simulink model "Project_PeregrineFalconDive_I"  (R2020b)
settings: Solver=VariableStepAuto  StartTime=0.0  StopTime=10.0  RelTol=1e-3
StartFcn:
  | learning.simulink.clearGlows(gcs);learning.simulink.resetGraderBadge(gcs);learning.simulink.closeNotificationBar(gcs);learning.simulink.Application.getInstance().clearStateflowBreakpoints()
StopFcn:
  | save_system(gcs);learning.simulink.refreshSignalWindows
model workspace (MAT data in the model file):
  courseObject.course = 'simulink'
  courseObject.chapter = 13
  courseObject.lesson = 1
  courseObject.section = 2
  courseObject.task = 1
undefined symbols (not defined in the file): A, Cd, g, m, rho
CloseFcn:
  | learning.simulink.cleanupOnlineTraining
settings Model: Creator=bhuva  LastModifiedBy=bhuva
settings DataIOCC: SaveTime=off

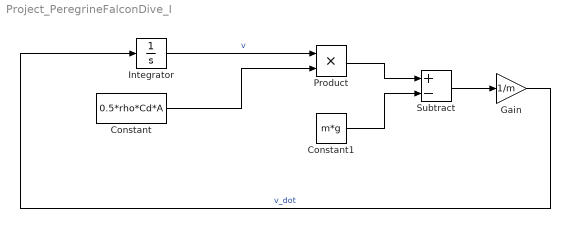
== system Project_PeregrineFalconDive_I ==
  Constant : Constant  Value=0.5*rho*Cd*A
  Constant1 : Constant  Value=m*g
  Gain : Gain  Gain=1/m
  Integrator : Integrator  InitialCondition=-10
  Product : Product
  Subtract : Sum  Inputs=+-
  wires:
  Integrator/1 -> Product/1  "v"
  Gain/1 -> Integrator/1  "v_dot"
  Constant/1 -> Product/2
  Product/1 -> Subtract/1
  Constant1/1 -> Subtract/2
  Subtract/1 -> Gain/1
